simulink model "AFS_ESP_rho"  (R2023a)
settings: Solver=FixedStepAuto  StartTime=0.0  StopTime=30.0  RelTol=1e-3
libraries: autolibshared x2
settings Model: Creator=ashkan  LastModifiedBy=ashkan

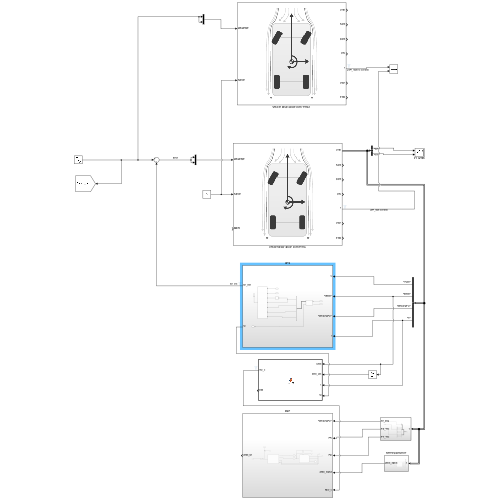
[thumbnail: Simulink's stored preview of the top-level diagram]
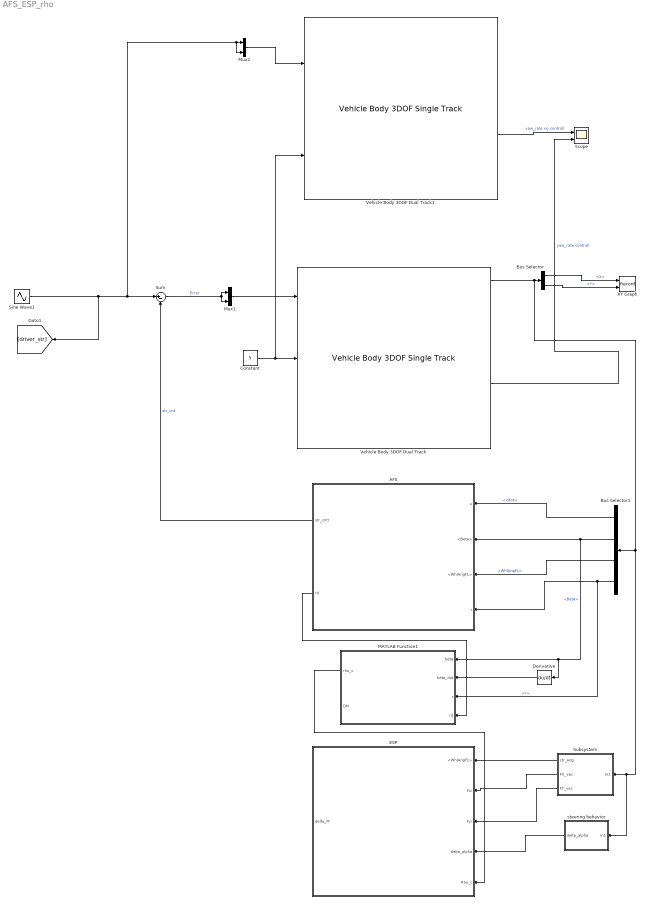
== system AFS_ESP_rho ==
  AFS : Subsystem
  Bus Selector : BusSelector  OutputSignals=InertFrm.Cg.Disp.X,InertFrm.Cg.Disp.Y
  Bus Selector1 : BusSelector  OutputSignals=BdyFrm.Cg.Vel.xdot,BdyFrm.Cg.Ang.Beta,BdyFrm.FrntAxl.Steer.WhlAngFL,BdyFrm.Cg.AngVel.r
  Constant : Constant  Value=5
  Derivative : Derivative
  ESP : Subsystem
  MATLAB Function1 : MATLAB Function  TreatAsAtomicUnit=on
  Mux1 : Mux  Inputs=2
  Mux2 : Mux  Inputs=2
  Scope : Scope  NumInputPorts=2
  Sine Wave1 : Sin  SampleTime=0
  Subsystem : Subsystem
  Sum : Sum  Inputs=|+-
  Vehicle Body 3DOF Dual Track : autolibshared/Vehicle Body 3DOF Single Track  trackMode=Dual  inputMode=External longitudinal velocity  frontSteerMode=on  rearSteerMode=off  windMode=off  muMode=off  extFMode=off  extMMode=on  htchFMode=off  htchMMode=off  extXo=off  extpsio=off  extxdoto=off  extro=off  extYo=off  extTamb=off  extydoto=off  aMode=2  NF=2  NR=2  m=2000  a=1.4  b=1.6  h=0.35  dh=1  hh=0.2  X_o=0  xdot_o=0  CalphaMode=off  sigmaMode=on  d=0  hl=0  w=[1.4,1.4]  Cy_f=12e3  Cy_r=11e3  sigma_f=.1  sigma_r=.1  alpha_f_brk=[-.1 .1]  Cy_f_data=[-9e3 9e3]  alpha_r_brk=[-.1 .1]  Cy_r_data=[-9e3 9e3]  Y_o=0  ydot_o=0  Izz=4000  psi_o=0  r_o=0  Af=2  Cd=.3  Cl=.1  Cpm=.1  beta_w=[0 0.01:0.01:0.3]  Cs=[0:0.03:0.9]  Cym=[0 1e-6:0.01:0.3]  Pabs=101325  Tair=273  g=9.81  mu=1  xdot_tol=.01  Fznom=5000  Fxtire_sat=7e4  Fytire_sat=7e4  longOff=0  latOff=0  vertOff=0  wrapAng=off
      settings: LibrarySourceBlock=vehdynlibeom/Vehicle Body 3DOF Dual Track
  Vehicle Body 3DOF Dual Track1 : autolibshared/Vehicle Body 3DOF Single Track  trackMode=Dual  inputMode=External longitudinal velocity  frontSteerMode=on  rearSteerMode=off  windMode=off  muMode=off  extFMode=off  extMMode=off  htchFMode=off  htchMMode=off  extXo=off  extpsio=off  extxdoto=off  extro=off  extYo=off  extTamb=off  extydoto=off  aMode=2  NF=2  NR=2  m=2000  a=1.4  b=1.6  h=0.35  dh=1  hh=0.2  X_o=0  xdot_o=0  CalphaMode=off  sigmaMode=on  d=0  hl=0  w=[1.4,1.4]  Cy_f=12e3  Cy_r=11e3  sigma_f=.1  sigma_r=.1  alpha_f_brk=[-.1 .1]  Cy_f_data=[-9e3 9e3]  alpha_r_brk=[-.1 .1]  Cy_r_data=[-9e3 9e3]  Y_o=0  ydot_o=0  Izz=4000  psi_o=0  r_o=0  Af=2  Cd=.3  Cl=.1  Cpm=.1  beta_w=[0 0.01:0.01:0.3]  Cs=[0:0.03:0.9]  Cym=[0 1e-6:0.01:0.3]  Pabs=101325  Tair=273  g=9.81  mu=1  xdot_tol=.01  Fznom=5000  Fxtire_sat=7e4  Fytire_sat=7e4  longOff=0  latOff=0  vertOff=0  wrapAng=off
      settings: LibrarySourceBlock=vehdynlibeom/Vehicle Body 3DOF Dual Track
  XY Graph : Record  FileSettingsInternal="{\"entries\":[{\"content\":{\"excelSettings\":{\"content\":{},\"type\":\"Streamout.ExcelSettings\"}},\"type\":\"Streamout.FileSettingStorage\",\"uuid\":\"\"}],\"packageUris\":[\"http:\\/\\/schema.mathworks.com\\/mf0\\/streamout_blocks\\/R2020a\"],\"version\":\"1.0\"}"  Layout=[1 1]  SignalsInternal="{\"entries\":[{\"content\":{\"signals\":[{\"content\":{\"blockPath\":[],\"dimensions\":[1],\"domain\":\"\",\"lineColor\":\"#a2142f\",\"plots\":[1],\"port\":1,\"sid\":[\"\"],\"signalID\":61071,\"signalName\":\"<X>\"},\"type\":\"RecordBlkView.Signal\",\"uuid\":\"\"},{\"content\":{\"blockPath\":[],\"dimensions\":[1],\"domain\":\"\",\"lineColor\":\"#139fff\",\"plots\":[1],\"port\":2,\"sid\":[\"\"],\"signalID\":61075,\"signalName\":\"<Y>\"},\"type\":\"RecordBlkView.Signal\",\"uuid\":\"\"}]},\"type\":\"RecordBlkView.InputSignals\",\"uuid\":\"\"}],\"packageUris\":[\"http:\\/\\/schema.mathworks.com\\/mf0\\/streamout_blocks\\/R2020a\"],\"version\":\"1.0\"}"  VisualizationBindings="{\"xyplotplugin\":{\"info\":[{\"series\":[{\"bindingParametersList\":[{\"parameter\":\"X-Axis\",\"signalID\":61071,\"signalName\":\"<X>\"},{\"parameter\":\"Y-Axis\",\"signalID\":61075,\"signalName\":\"<Y>\"}],\"seriesID\":48603}],\"subplotID\":1}]}}"  CompatibilityTag=XY
  steering behavior : Subsystem
  wires:
  Mux1/1 -> Vehicle Body 3DOF Dual Track/1
  Sum/1 -> Mux1/2, Mux1/1  "Error"
  Sine Wave1/1 -> [driver_str], Mux2/2, Mux2/1, Sum/1
  MATLAB Function1/1(rho_c) -> ESP/5(Rho_c)
  Vehicle Body 3DOF Dual Track/5 -> Scope/2  "yaw_rate controll"
  Bus Selector/1 -> XY Graph/1  "<X>"
  Bus Selector/2 -> XY Graph/2  "<Y>"
  Constant/1 -> Vehicle Body 3DOF Dual Track1/2, Vehicle Body 3DOF Dual Track/2
  Bus Selector1/1 -> AFS/1(u)  "<xdot>"
  Bus Selector1/2 -> AFS/2(<Beta>), Derivative/1, MATLAB Function1/1(beta)  "<Beta>"
  Bus Selector1/3 -> AFS/3(<WhlAngFL>)  "<WhlAngFL>"
  Bus Selector1/4 -> MATLAB Function1/3(r), AFS/4(r)  "<r>"
  Derivative/1 -> MATLAB Function1/2(beta_dot)
  AFS/2(rd) -> MATLAB Function1/4(rd)
  Vehicle Body 3DOF Dual Track/1 -> steering behavior/1(In1), Subsystem/1(In1), Bus Selector1/1, Bus Selector/1
  Subsystem/1(str_ang) -> ESP/1(<WhlAngFL>)
  Subsystem/2(FX_vec) -> ESP/2(Fxi)
  steering behavior/1(delta_alpha) -> ESP/4(delta_alpha)
  Subsystem/3(FY_vec) -> ESP/3(Fyi)
  Mux2/1 -> Vehicle Body 3DOF Dual Track1/1
  Vehicle Body 3DOF Dual Track1/5 -> Scope/1  "yaw_rate no controll"
  AFS/1(str_cntr) -> Sum/2  "str_cnt"

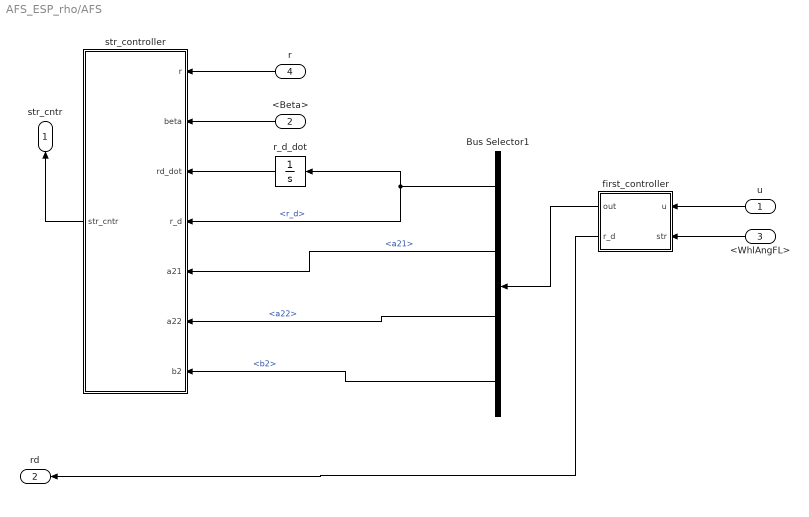
== system AFS_ESP_rho/AFS ==
  u : Inport
  <Beta> : Inport  Port=2
  <WhlAngFL> : Inport  Port=3
  r : Inport  Port=4
  Bus Selector1 : BusSelector  OutputSignals=r_d,a21,a22,b2
  first_controller : MATLAB Function  TreatAsAtomicUnit=on
  r_d_dot : Integrator
  str_controller : MATLAB Function  TreatAsAtomicUnit=on
  str_cntr : Outport
  rd : Outport  Port=2
  wires:
  <Beta>/1 -> str_controller/2(beta)
  r/1 -> str_controller/1(r)
  first_controller/1(out) -> Bus Selector1/1
  <WhlAngFL>/1 -> first_controller/2(str)
  u/1 -> first_controller/1(u)
  Bus Selector1/2 -> str_controller/5(a21)  "<a21>"
  Bus Selector1/3 -> str_controller/6(a22)  "<a22>"
  str_controller/1(str_cntr) -> str_cntr/1
  r_d_dot/1 -> str_controller/3(rd_dot)
  Bus Selector1/1 -> str_controller/4(r_d), r_d_dot/1  "<r_d>"
  Bus Selector1/4 -> str_controller/7(b2)  "<b2>"
  first_controller/2(r_d) -> rd/1

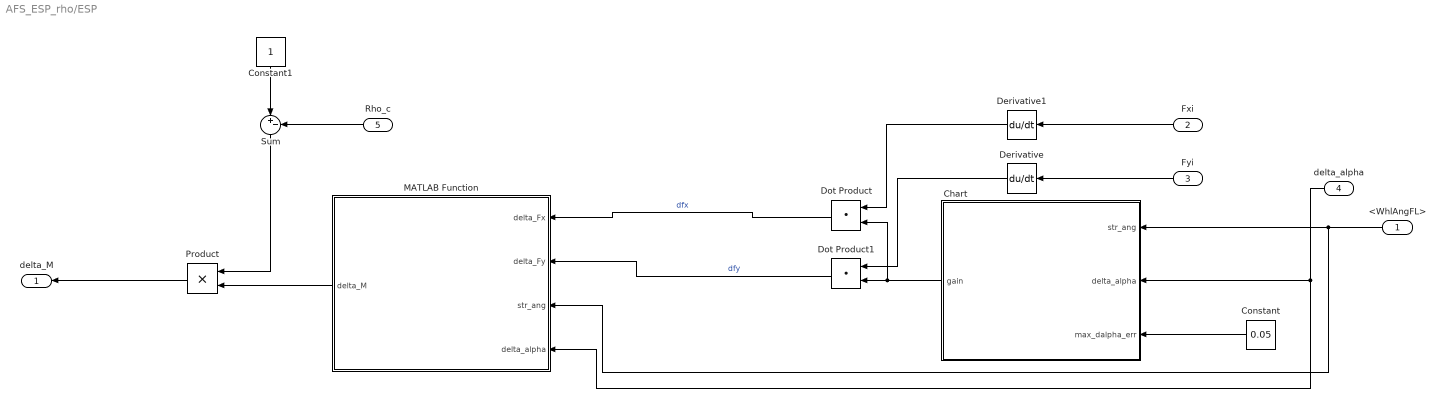
== system AFS_ESP_rho/ESP ==
  <WhlAngFL> : Inport
  Fxi : Inport  Port=2
  Fyi : Inport  Port=3
  delta_alpha : Inport  Port=4
  Rho_c : Inport  Port=5
  Chart : Stateflow chart  TreatAsAtomicUnit=on
  Constant : Constant  Value=0.05
  Constant1 : Constant
  Derivative : Derivative
  Derivative1 : Derivative
  Dot Product : DotProduct  OutDataTypeStr=Inherit: Inherit via internal rule
  Dot Product1 : DotProduct  OutDataTypeStr=Inherit: Inherit via internal rule
  MATLAB Function : MATLAB Function  TreatAsAtomicUnit=on
  Product : Product
  Sum : Sum  Inputs=|+-
  delta_M : Outport
  wires:
  <WhlAngFL>/1 -> MATLAB Function/3(str_ang), Chart/1(str_ang)
  Constant/1 -> Chart/3(max_dalpha_err)
  Chart/1(gain) -> Dot Product1/2, Dot Product/2
  Fxi/1 -> Derivative1/1
  Fyi/1 -> Derivative/1
  Derivative1/1 -> Dot Product/1
  Dot Product/1 -> MATLAB Function/1(delta_Fx)  "dfx"
  Derivative/1 -> Dot Product1/1
  Dot Product1/1 -> MATLAB Function/2(delta_Fy)  "dfy"
  MATLAB Function/1(delta_M) -> Product/2
  delta_alpha/1 -> Chart/2(delta_alpha), MATLAB Function/4(delta_alpha)
  Rho_c/1 -> Sum/2
  Constant1/1 -> Sum/1
  Sum/1 -> Product/1
  Product/1 -> delta_M/1

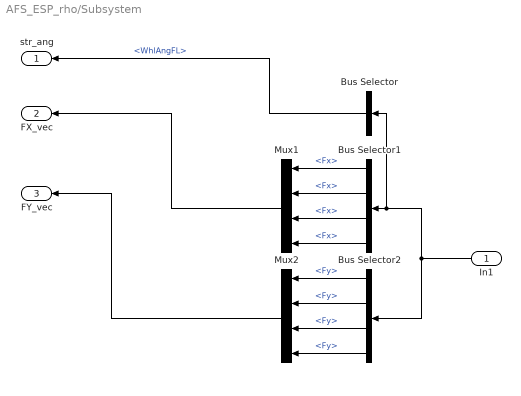
== system AFS_ESP_rho/Subsystem ==
  In1 : Inport
  Bus Selector : BusSelector  OutputSignals=BdyFrm.FrntAxl.Steer.WhlAngFL
  Bus Selector1 : BusSelector  OutputSignals=BdyFrm.Forces.FrntAxl.Lft.Fx,BdyFrm.Forces.FrntAxl.Rght.Fx,BdyFrm.Forces.RearAxl.Lft.Fx,BdyFrm.Forces.RearAxl.Rght.Fx
  Bus Selector2 : BusSelector  OutputSignals=BdyFrm.Forces.FrntAxl.Lft.Fy,BdyFrm.Forces.FrntAxl.Rght.Fy,BdyFrm.Forces.RearAxl.Lft.Fy,BdyFrm.Forces.RearAxl.Rght.Fy
  Mux1 : Mux
  Mux2 : Mux
  str_ang : Outport
  FX_vec : Outport  Port=2
  FY_vec : Outport  Port=3
  wires:
  Mux1/1 -> FX_vec/1
  Bus Selector1/4 -> Mux1/4  "<Fx>"
  In1/1 -> Bus Selector2/1, Bus Selector/1, Bus Selector1/1
  Bus Selector2/4 -> Mux2/4  "<Fy>"
  Bus Selector1/2 -> Mux1/2  "<Fx>"
  Mux2/1 -> FY_vec/1
  Bus Selector1/3 -> Mux1/3  "<Fx>"
  Bus Selector2/3 -> Mux2/3  "<Fy>"
  Bus Selector2/1 -> Mux2/1  "<Fy>"
  Bus Selector2/2 -> Mux2/2  "<Fy>"
  Bus Selector1/1 -> Mux1/1  "<Fx>"
  Bus Selector/1 -> str_ang/1  "<WhlAngFL>"

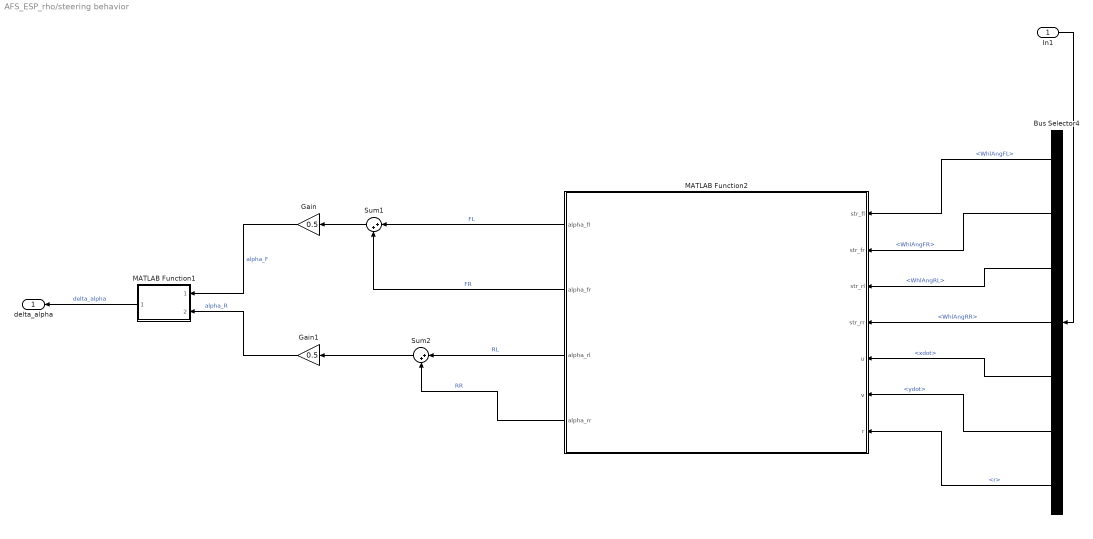
== system AFS_ESP_rho/steering behavior ==
  In1 : Inport
  Bus Selector4 : BusSelector  OutputSignals=BdyFrm.FrntAxl.Steer.WhlAngFL,BdyFrm.FrntAxl.Steer.WhlAngFR,BdyFrm.RearAxl.Steer.WhlAngRL,BdyFrm.RearAxl.Steer.WhlAngRR,BdyFrm.Cg.Vel.xdot,BdyFrm.Cg.Vel.ydot,BdyFrm.Cg.AngVel.r
  Gain : Gain  Gain=0.5
  Gain1 : Gain  Gain=0.5
  MATLAB Function1 : MATLAB Function  TreatAsAtomicUnit=on
  MATLAB Function2 : MATLAB Function  TreatAsAtomicUnit=on
  Sum1 : Sum  Inputs=|++
  Sum2 : Sum  Inputs=|++
  delta_alpha : Outport
  wires:
  MATLAB Function1/1(delta_alpha) -> delta_alpha/1  "delta_alpha"
  In1/1 -> Bus Selector4/1
  MATLAB Function2/3(alpha_rl) -> Sum2/1  "RL"
  Sum1/1 -> Gain/1
  MATLAB Function2/2(alpha_fr) -> Sum1/2  "FR"
  MATLAB Function2/1(alpha_fl) -> Sum1/1  "FL"
  Bus Selector4/5 -> MATLAB Function2/5(u)  "<xdot>"
  Bus Selector4/3 -> MATLAB Function2/3(str_rl)  "<WhlAngRL>"
  Sum2/1 -> Gain1/1
  Gain/1 -> MATLAB Function1/1(alpha_f)  "alpha_F"
  Gain1/1 -> MATLAB Function1/2(alpha_r)  "alpha_R"
  Bus Selector4/1 -> MATLAB Function2/1(str_fl)  "<WhlAngFL>"
  Bus Selector4/6 -> MATLAB Function2/6(v)  "<ydot>"
  Bus Selector4/7 -> MATLAB Function2/7(r)  "<r>"
  MATLAB Function2/4(alpha_rr) -> Sum2/2  "RR"
  Bus Selector4/2 -> MATLAB Function2/2(str_fr)  "<WhlAngFR>"
  Bus Selector4/4 -> MATLAB Function2/4(str_rr)  "<WhlAngRR>"

== matlab function AFS_ESP_rho/steering behavior/MATLAB Function1 ==
  data: alpha_f input; delta_alpha output; alpha_r input
function delta_alpha = fcn(alpha_f , alpha_r)

delta_alpha = alpha_r - alpha_f;

== matlab function AFS_ESP_rho/steering behavior/MATLAB Function2 ==
  data: str_fl input; str_fr input; str_rl input; str_rr input; u input; alpha_fl output; v input; r input; alpha_fr output; alpha_rl output; alpha_rr output; vehicle_data parameter
function [alpha_fl , alpha_fr , alpha_rl , alpha_rr] = fcn(str_fl , str_fr , str_rl , str_rr , u , v , r , vehicle_data)


    a = vehicle_data.vehicle.Lf;
    b = vehicle_data.vehicle.Lr;
    Tw = vehicle_data.vehicle.Wf;
    
    alpha_fl = str_fl - atan((v+ a*r )/(u + 0.5*Tw*r ));
    alpha_fr = str_fr - atan((v+ a*r )/(u - 0.5*Tw*r ));
    alpha_rl = str_rl + atan((b*r - v )/(u + 0.5*Tw*r ));
    alpha_rr = str_rr + atan((b*r - v )/(u - 0.5*Tw*r ));


end

== matlab function AFS_ESP_rho/AFS/first_controller ==
  data: out output Bus: out_rd_bus; u input; str input; vehicle_data parameter; r_d output
function [out, r_d] = r_d(u , str, vehicle_data)


% here is some simplified parameters :)
   m = vehicle_data.vehicle.m;
   a = vehicle_data.vehicle.Lf;
   b = vehicle_data.vehicle.Lr;
   izz = vehicle_data.vehicle.i_zz;
   g = vehicle_data.vehicle.g;
   L = vehicle_data.vehicle.L;
   mu = vehicle_data.AFS.mu;  % --> should come from scenario
   Caf = vehicle_data.front_suspension.Ks_f ;
   Car = vehicle_data.rear_suspension.Ks_r;
   
   
% lets calculate some live parameters!!! _|_
    
   r_up_lim = 0.85 * abs(mu*g / u);
   r_ss = (2*L*Caf*Car*u)/(2*Car*Caf*L^2 - m*u^2*(a*Caf - b*Car)) * str;
   r_d = min(r_ss , r_up_lim)* sign(str);
 
   a11 = (-2*Caf - 2*Car)/(m * u);
   a12 = -1 + (2*Car*b - 2*Caf*a)/(m * u^2);
   a21 = (2*Car*b - 2*Caf*a)/izz;
   a22 = (-2*Caf*a^2 - 2*Car*b^2)/(izz * u);
   b1 = (2*Caf)/(m * u);
   b2 = (2 * Caf * a)/izz;

% outputs
   out.a11 = a11;
   out.a21 = a21;
   out.a12 = a12;
   out.a22 = a22;
   out.b1 = b1;
   out.b2 = b2;
   out.r_d = r_d;

end

== matlab function AFS_ESP_rho/AFS/str_controller ==
  data: r input; beta input; rd_dot input; r_d input; a21 input; str_cntr output; a22 input; b2 input; vehicle_data parameter
function str_cntr = str_controller(r, beta , rd_dot , r_d , a21 , a22 , b2, vehicle_data)

%    lambda = AFS.lambda;
    s = r - r_d;
    lambda = vehicle_data.AFS.lambda;
    X      = vehicle_data.AFS.X;
    str_cntr = ((1/b2) * (-a21*beta - a22*r + rd_dot - lambda*(r - r_d))) - sign(s)*X;


end

== matlab function AFS_ESP_rho/MATLAB Function1 ==
  data: rho_c output; beta input; beta_dot input; r input; rd input; DM output; vehicle_data parameter
function [rho_c , DM] = rho_C(beta , beta_dot , r ,rd, vehicle_data)
    
    k1 = vehicle_data.AFS.k1;
    k2 = vehicle_data.AFS.k2;
    B1 = vehicle_data.AFS.B1;
    B2 = vehicle_data.AFS.B2;

    
    if abs(k1*beta_dot + k2*beta) < B1
        rho_c = 1;
    elseif abs(k1*beta_dot + k2*beta) > B2
        rho_c = 0;
    else
        rho_c = (B2 - abs(k1*beta_dot + k2*beta))/(B2 - B1);
    end
    
    DM_z = (1-rho_c)*(k1*abs(r-rd) - k2*abs(beta));
    DM_x = 0;
    DM_y = 0;

    DM = [DM_x , DM_y , DM_z];
end

== stateflow chart AFS_ESP_rho/ESP/Chart ==
  state ESP_ON
    state FRONT_WHEEL
      state FRONT_LEFT
        gain = [1 0 0 0];
      state FRONT_RIGHT
        gain = [0 1 0 0] ;
      (junction 36) -> FRONT_LEFT [order 2] : [str_ang <0]
      (junction 36) -> FRONT_RIGHT [order 1] : [str_ang >     0]
      FRONT_RIGHT -> (junction 36)
      FRONT_LEFT -> (junction 36)
    state REAR_WHEEL
      state REAR_LEFT
        gain = [0 0 1 0];
      state REAR_RIGHT
        gain = [0 0 0 1];
      (junction 38) -> REAR_LEFT [order 1] : [str_ang > 0]
      (junction 38) -> REAR_RIGHT [order 2] : [str_ang < 0]
      REAR_RIGHT -> (junction 38)
      REAR_LEFT -> (junction 38)
    (junction 31) -> (junction 36) [order 1] : [delta_alpha > 0 ]
    FRONT_WHEEL -> (junction 31)
    REAR_WHEEL -> (junction 31)
    (junction 31) -> (junction 38) [order 2] : [delta_alpha < 0]
  state ESP_OFF
    gain = [0 0 0 0]   ;
  (default) -> ESP_OFF
  ESP_OFF -> (junction 31) : [ abs(delta_alpha) > max_dalpha_err + 0.01   ]
  ESP_ON -> ESP_OFF : [abs(delta_alpha  ) < max_dalpha_err - 0.01]
  data: str_ang input; delta_alpha input; max_dalpha_err input; gain output

== matlab function AFS_ESP_rho/ESP/MATLAB Function ==
  data: delta_Fx input; delta_M output; delta_Fy input; str_ang input; delta_alpha input; vehicle_data parameter
function delta_M   = yaw_moment_diff(delta_Fx , delta_Fy ,  str_ang , delta_alpha , vehicle_data)

    a = vehicle_data.vehicle.Lf;
    b = vehicle_data.vehicle.Lr;
    L = vehicle_data.vehicle.L;
    Tw = vehicle_data.vehicle.Wf;

    if delta_alpha > 0      % over steering

    
        delta_Mz = (delta_Fx*(0.5*Tw*cos(str_ang) + a*sin(str_ang))) - (delta_Fy * (a*cos(str_ang) - 0.5*Tw*sin(str_ang)));

        
    elseif delta_alpha < 0  % under steering

        
        delta_Mz = (delta_Fx * 0.5*Tw) - (delta_Fy * b);

    else    % natural steering
        delta_Mz = 0;

    end

    delta_Mx = 0;

    delta_My = 0;

    delta_M = [delta_Mx , delta_My , delta_Mz];

end
